simulink library "HY_General_Library"  (R2018b)
settings: Solver=ode45  StartTime=0.0  StopTime=10.0  RelTol=1e-3  EnableMultiTasking=on
undefined symbols (not defined in the file or in its folder): dT, Slope1, Slope2
libraries: simulink x63, $bdroot x4
(part 1 of 5)
settings Model: Creator=zhangzhi35  LastModifiedBy=xuhongjiang01
settings DataIOCC: LimitDataPoints=on  SaveFormat=Array
settings OptimizationCC: LifeSpan=inf
settings DebuggingCC: SolverPrmCheckMsg=warning  SFUnexpectedBacktrackingDiag=warning  SFNoUnconditionalDefaultTransitionDiag=warning  SFExecutionAtInitializationDiag=none
settings HardwareCC: ProdBitPerPointer=32  ProdBitPerSizeT=32  ProdBitPerPtrDiffT=32  ProdLargestAtomicFloat=None  ProdIntDivRoundTo=Undefined  ProdEndianess=Unspecified  ProdWordSize=32  ProdHWDeviceType=32-bit Generic
settings ModelReferenceCC: PropagateSignalLabelsOutOfModel=off
settings SFSimCC: SimUseLocalCustomCode=off
settings RTWCC: RTWUseLocalCustomCode=off
settings CodeAppCC: StateflowObjectComments=on
settings GRTTargetCC: TargetLangStandard=C89/C90 (ANSI)  GeneratePreprocessorConditionals=Disable all
settings ConfigComp: CovMetricSettings=dw  CovHtmlReporting=on  CovSaveCumulativeToWorkspaceVar=on  CovSaveSingleToWorkspaceVar=on  CovExternalEMLEnable=off  CovSFcnEnable=off

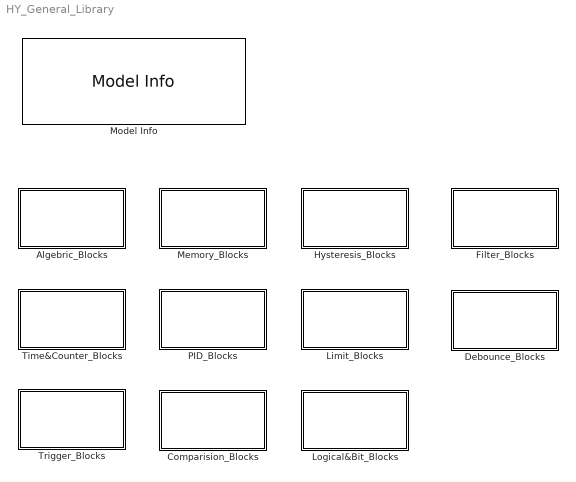
== system HY_General_Library ==
  Algebric_Blocks : Subsystem
      mask Display:
      | color('magenta')
      | fprintf('ALGEBRIC\nBLOCKS')
  Comparision_Blocks : Subsystem
      mask Display:
      | color('magenta')
      | fprintf('COMPARISION\nBLOCKS')
  Debounce_Blocks : Subsystem
      mask Display:
      | color('magenta')
      | fprintf('DEBOUNCE\nBLOCKS')
  Filter_Blocks : Subsystem
      mask Display:
      | color('magenta')
      | fprintf('FILTER\nBLOCKS')
  Hysteresis_Blocks : Subsystem
      mask Display:
      | color('magenta')
      | fprintf('HYSTERESIS\nBLOCKS')
  Limit_Blocks : Subsystem
      mask Display:
      | color('magenta')
      | fprintf('LIMIT\nBLOCKS')
  Logical&Bit_Blocks : Subsystem
      mask Display:
      | color('magenta')
      | fprintf('LOGIC&BIT\nBLOCKS')
  Memory_Blocks : Subsystem
      mask Display:
      | color('magenta')
      | fprintf('MEMORY\nBLOCKS')
  Model Info : simulink/Model-Wide Utilities/Model Info  Frame=on  DisplayStringWithTags=|  HorizontalTextAlignment=Left  LeftAlignmentValue=0.02
      | ModelName:     %<ModelName>                   
      |   Creator:             %<Creator>
      |   Created Date:   %<Created>
      |   ModelVersion:   %<ModelVersion>
      |   LastModifier:     %<LastModifiedBy>
      |   Modified Date:   %<LastModificationDate>
  PID_Blocks : Subsystem
      mask Display:
      | color('magenta')
      | fprintf('PID\nBLOCKS')
  Time&Counter_Blocks : Subsystem
      mask Display:
      | color('magenta')
      | fprintf('TIME&COUNTER\nBLOCKS')
  Trigger_Blocks : Subsystem
      mask Display:
      | color('magenta')
      | fprintf('TRIGGER\nBLOCKS')

== system HY_General_Library/Algebric_Blocks ==
  DIVIDE : Subsystem  mask(DIVIDE){MinRange=1e-5}
      mask prompts: MinRange "Smallest allowed value to divide by"
      mask help:
      | HY Library for Function Development
      |
      | Divides two inputs with divide by zero protection.
      |
      | The minimal value to divide by is set by the project lead and may not be changed.
      |
      | When abs(second input) is less than the specified MinRange,
      | then the second input is substituted by MinRange or -MinRange for negative values.
      mask init:
      | val=get_param(gcb,'MinRange');
      | if strcmp(val,'0')
      |     val = '1e-5';
      |     set_param(gcb,'MinRange',val);
      |     errordlg('Invalid setting in block DIVIDE_Protect');  
      | end
      mask Display:
      | port_label('input',1,'×');
      | port_label('input',2,'÷')
      | color('magenta');
      | text(1,0,'HY','horizontalAlignment','right','verticalAlignment','bottom');
  TrqPwr_Cnv : Subsystem  mask(TrqPwr_Cnv){CnvType=TrqSpd --> Pwr, Trq2Pwr=boolean(1)}
      mask prompts: CnvType "转换类型:"; Trq2Pwr "Mask Parameter 2:"
      mask help:
      | 皓耘功能开发库
      |
      | 扭矩功率转换器
      |
      | 可在参数设置界面选择转换类型
      | P=TN/9550
      |
      | 输入/输出：
      | Spd：转速信号，单位RPM
      | Trq：扭矩，单位Nm
      | Pwr：功率，单位kW
      mask Help:
      | 1、功率扭矩计算速度，使用公式 N = P * 9550 / T
      | 2、功率速度计算扭矩，使用公式 T = P * 9550 / N
      | 3、扭矩速度计算功率，使用公式 P = T * N / 9550
      | 
      | 1与2可使用同一类型计算
      mask TypeOptions CnvType: TrqSpd --> Pwr | PwrSpd --> Trq | PwrTrq --> Spd
      mask Callback CnvType:
      | switch get_param(gcb,'CnvType')
      |     case 'TrqSpd --> Pwr'
      |         Trq2Pwr = 1;
      |     case 'PwrSpd --> Trq'
      |         Trq2Pwr = 0;
      |     case 'PwrTrq --> Spd'
      |         Trq2Pwr = 0;
      | end
      | set_param(gcb,'Trq2Pwr',['boolean(' num2str(Trq2Pwr) ')']);
      mask Display:
      | port_label('input',1,CnvType(1:3));
      | port_label('input',2,CnvType(4:6));
      | port_label('output',1,CnvType(end-2:end));
      | color('blue')
      | disp(CnvType, 'texmode','on')
      | color('magenta');
      | text(1,0,'HY','horizontalAlignment','right','verticalAlignment','bottom');
  Unit_Cnv : Subsystem  RTWFcnName=Unit_Cnv  RTWFileName=SEN_MDL_LIB  mask(Unit conversions){CnvType=km/h --> m/s, g=single(0.27778)}
      mask prompts: CnvType "Conversion Type:"; g "Mask Parameter 2:"
      mask help:
      | 皓耘功能开发库
      |
      | Conversions of units.
      settings: RTWFcnNameOpts=User specified  RTWFileNameOpts=User specified
      mask TypeOptions CnvType: rad --> deg | deg --> rad | pascal --> bar | bar --> pascal | kilopascal --> bar | bar --> kilopascal | min --> sec | sec --> min | hour --> sec | sec --> hour | km --> mile | mile --> km | km/h --> m/s | m/s --> km/h | rad/s --> rpm | rpm --> rad/s | xx --> kiloxx | kiloxx --> xx
      mask Callback CnvType:
      | switch get_param(gcb,'CnvType')
      |     case 'rad --> deg'
      |         g = 57.2958;
      |     case 'deg --> rad'
      |         g = 0.017453;
      |     case 'bar --> pascal'
      |         g=1e5;
      |     case 'pascal --> bar'
      |         g=1e-5;
      |     case 'bar --> kilopascal'
      |         g=100;
      |     case 'kilopascal --> bar'
      |         g=0.01;
      |     case 'min --> sec'
      |         g=60;
      |     case 'sec --> min'
      |         g=1/60;
      |     case 'hour --> sec'
      |         g=3600;
      |     case 'sec --> hour'
      |         g=1/3600;
      |     case 'km --> mile'
      |         g=1/1.6093;
      |     case 'mile --> km'
      |         g=1.6093;
      |     case 'km/h --> m/s'
      |         g=1000/3600;
      |     case 'm/s --> km/h'
      |         g=3.6;
      |     case 'rad/s --> rpm'
      |         g=60/(2*pi);
      |     case 'rpm --> rad/s'
      |         g=2*pi/60;
      |     case 'xx --> kiloxx'
      |         g=0.001;
      |     case 'kiloxx --> xx'
      |         g=1000;
      | end
      | set_param(gcb,'g',['single(' num2str(g) ')']);
      mask Display:
      | color('blue')
      | disp(CnvType, 'texmode','on')
      | color('magenta');
      | text(0.93,0,'HY','horizontalAlignment','right','verticalAlignment','bottom');

== system HY_General_Library/Comparision_Blocks ==
  Open_Interval : Subsystem  RTWFcnName=Open_Interval  RTWFileName=SEN_MDL_LIB  mask(Open_Interval){CompareType=L<u<H, sIndex=uint8(0)}
      mask prompts: CompareType "Comparision Type:"; sIndex "Switch Parameter"
      mask help:
      | 皓耘功能开发库
      |
      | 区间模块
      |
      | 输入:
      | H：上限阀值
      | u：信号输入
      | L：下限阀值
      |
      | 输出：
      | y：输出信号（布尔型）
      settings: MinAlgLoopOccurrences=on  RTWFcnNameOpts=User specified  RTWFileNameOpts=User specified
      mask TypeOptions CompareType: L<u<H | L≤x<H | L<x≤H | L≤x≤H
      mask Callback CompareType:
      | switch get_param(gcb,'CompareType')
      |     case 'L<u<H'
      |         sIndex = 0;
      |     case 'L≤x<H'
      |         sIndex = 1;
      |     case 'L<x≤H'
      |         sIndex = 2;
      |     case 'L≤x≤H'
      |         sIndex = 3;
      | end
      | set_param(gcb,'sIndex',['uint8(' num2str(sIndex) ')']);
      mask Display:
      | color('blue');
      | disp(CompareType, 'texmode','on');
      | color('black');
      | port_label('input',1,'H');
      | port_label('input',2,'u');
      | port_label('input',3,'L');
      | color('orange');
      | port_label('output',1,'y');
      | color('magenta');
      | text(1,0,'HY','horizontalAlignment','right','verticalAlignment','bottom');

== system HY_General_Library/Debounce_Blocks ==
  DebounceB : Subsystem  RTWFcnName=Debounce  RTWFileName=SEN_MDL_LIB  mask(DebounceB){InitialValue=0}
      mask prompts: InitialValue "初始输出值"
      mask help:
      | 皓耘功能开发库
      |
      | 开关信号防抖模块
      |
      | 输入：
      | u：     开关信号输入（布尔型）
      | TAct：  Active确认时间（浮点类型）
      | TDeact：Deactive激活确认时间（浮点类型）
      | dT：    模块运行单步时间（浮点类型）
      |
      | 输出：
      | y：     防抖处理后输出信号（布尔型）
      mask init:
      | val = get_param(gcb,'InitialValue');
      | if strcmp(val,'0')==0 && strcmp(val,'1')==0
      |     val = '0';
      |     set_param(gcb,'InitialValue',val);
      |     errordlg('This parameter can only be set to 0 or 1');  
      | end
      settings: RTWFcnNameOpts=User specified  RTWFileNameOpts=User specified
      mask Display:
      | color('orange');
      | port_label('input',1,'u');
      | port_label('output',1,'y');
      | color('black');
      | port_label('input',2,'TAct');
      | port_label('input',3,'TDeact');
      | port_label('input',4,'dT');
      | 
      | color('red')
      | plot([0.10 0.20 0.20],[0.55 0.55 0.75])
      | plot([0.20 0.22 0.22],[0.75 0.75 0.55])
      | plot([0.22 0.24 0.24],[0.55 0.55 0.75])
      | plot([0.24 0.26 0.26],[0.75 0.75 0.55])
      | plot([0.26 0.28 0.28],[0.55 0.55 0.75])
      | plot([0.28 0.70 0.70],[0.75 0.75 0.55])
      | plot([0.70 0.72 0.72],[0.55 0.55 0.75])
      | plot([0.72 0.74 0.74],[0.75 0.75 0.55])
      | plot([0.74 0.76 0.76],[0.55 0.55 0.75])
      | plot([0.76 0.78 0.78 0.90],[0.75 0.75 0.55 0.55])
      | plot([0.10 0.28 0.28],[0.25 0.25 0.45])
      | plot([0.28 0.78 0.78 0.90],[0.45 0.45 0.25 0.25])
      | color('black')
      | plot([0.20 0.27],[0.55 0.75])
      | plot([0.20 0.27],[0.75 0.55])
      | plot([0.70 0.78],[0.55 0.75])
      | plot([0.70 0.78],[0.75 0.55])
      | color('blue')
      | text(0.35,0.1,sprintf('InitVal=%s', char(val)));
      | color('magenta')
      | text(1,0,'HY','horizontalAlignment','right','verticalAlignment','bottom')
  DebounceJump : Subsystem  mask(DebounceJump){}
      mask help:
      | 皓耘功能开发库
      |
      | 信号跳变处理模块
      |
      | 输入信号与上一时刻输出值相差超过设定幅值开始计时，否则计时清零
      | 计时超过最大检查时间，输出当前值，否则，输出上一时刻值
      |
      | 输入：
      | u：    需处理信号
      | Thd：  信号跳变幅值
      | ChkTi：最大检查时间（秒）
      | dT：   模块运行单步时间（秒）
      |
      | 输出：
      | y：    处理后的信号
      mask Display:
      | color('magenta');
      | text(1,0,'HY','horizontalAlignment','right','verticalAlignment','bottom');
  Debounce_Cnt : Subsystem  RTWFcnName=Debounce  RTWFileName=SEN_MDL_LIB  mask(Debounce_Cnt){InitialValue=0}
      mask prompts: InitialValue "初始输出值"
      mask help:
      | 皓耘功能开发库
      |
      | 基于运行次数的开关信号防抖模块
      |
      | 输入：
      | u：     开关信号输入（布尔型）
      | ONCnt： ON延时次数（无符号整型）
      | OFFCnt：ON延时次数（无符号整型）
      |
      | 输出：
      | y：     防抖处理后输出信号（布尔型）
      mask init:
      | val = get_param(gcb,'InitialValue');
      | if strcmp(val,'0')==0 && strcmp(val,'1')==0
      |     val = '0';
      |     set_param(gcb,'InitialValue',val);
      |     errordlg('This parameter can only be set to 0 or 1');  
      | end
      settings: RTWFcnNameOpts=User specified  RTWFileNameOpts=User specified
      mask Display:
      | color('orange');
      | port_label('input',1,'u');
      | port_label('output',1,'y');
      | color('black');
      | port_label('input',2,'ONCnt');
      | port_label('input',3,'OFFCnt');
      | 
      | color('red')
      | plot([0.10 0.20 0.20],[0.55 0.55 0.75])
      | plot([0.20 0.22 0.22],[0.75 0.75 0.55])
      | plot([0.22 0.24 0.24],[0.55 0.55 0.75])
      | plot([0.24 0.26 0.26],[0.75 0.75 0.55])
      | plot([0.26 0.28 0.28],[0.55 0.55 0.75])
      | plot([0.28 0.70 0.70],[0.75 0.75 0.55])
      | plot([0.70 0.72 0.72],[0.55 0.55 0.75])
      | plot([0.72 0.74 0.74],[0.75 0.75 0.55])
      | plot([0.74 0.76 0.76],[0.55 0.55 0.75])
      | plot([0.76 0.78 0.78 0.90],[0.75 0.75 0.55 0.55])
      | plot([0.10 0.28 0.28],[0.25 0.25 0.45])
      | plot([0.28 0.78 0.78 0.90],[0.45 0.45 0.25 0.25])
      | color('black')
      | plot([0.20 0.27],[0.55 0.75])
      | plot([0.20 0.27],[0.75 0.55])
      | plot([0.70 0.78],[0.55 0.75])
      | plot([0.70 0.78],[0.75 0.55])
      | color('blue')
      | text(0.35,0.1,sprintf('InitVal=%s', char(val)));
      | color('magenta')
      | text(1,0,'HY','horizontalAlignment','right','verticalAlignment','bottom')
  Debounce_OBD_FCN : Subsystem  TreatAsAtomicUnit=on  mask(Debounce_OBD_FCN){}
      mask help:
      | 皓耘功能开发库
      |
      | ISO 14229 D.5  DTC-FaultDetectionCounter operation definition
      | 输入：
      | bErr        Error signal(s)  (i.e. vector of continuous test runs)
      | bRst        Reset flag  (true/false)
      | bEna        Enable flag (true/false)
      | FailThd     counter a value between 0 and 32767  (for each bErr signal)
      | RecThd      counter a value between 0 and -32768 (for each bErr signal)
      | IncrFail    increment Fault counter (>0) max 255 in timer ticks for each signal
      | DecrRec     decrement Recovery counter (<0) min -128 in timer ticks for each
      |             signal
      |
      | So Counters are in numbers of timer ticks of tiTaskA(=0.01);
      | E.g. if Increment counter is 5 and decrement counter -3 then
      | maximum fail and recovery times are:
      | 32767*0.01/5 = 65.534 sec and -32768*0.01/3 = 109.2267 sec at most
      |
      | Outputs :
      | bFailed testFailed  (Bit 0)
      |
      | Notes:
      | * Outputs are held when input bEna is disabled
      | * Due to Int16 instead of Int8 and Incr/Decr 5/-3 by default the above
      | mentioned ISO standard is somewhat changed.
      mask Display:
      | color('black');
      | plot([0.2,0.2],[0.1,0.9]);
      | plot([0.205,0.205],[0.1,0.9]);
      | plot([0.2,0.8],[0.8,0.8]);
      | plot([0.2,0.8],[0.65,0.65]);
      | plot([0.2,0.8],[0.45,0.45]);
      | plot([0.2,0.8],[0.25,0.25]);
      | plot([0.2,0.8],[0.1,0.1]);
      | port_label('input',1,'bErr');
      | port_label('input',2,'bRst');
      | port_label('input',3,'bEna');
      | port_label('input',4,'FailThd');
      | port_label('input',5,'RecThd');
      | port_label('input',6,'IncrFail');
      | port_label('input',7,'DecrRec');
      | port_label('output',1,'bFailed');
      | color('cyan');
      | plot([0.3,0.3],[0.1,0.9]);
      | plot([0.4,0.4],[0.1,0.9]);
      | plot([0.5,0.5],[0.1,0.9]);
      | color('orange');
      | plot([0.2,0.3,0.3,0.6,0.6,0.8],[0.85,0.85,0.8,0.8,0.85,0.85]);
      | plot([0.2,0.5,0.5,0.6,0.6,0.8],[0.7,0.7,0.65,0.65,0.7,0.7]);
      | color('blue');
      | plot([0.2,0.3,0.4,0.5,0.5,0.6,0.7,0.8],[0.45,0.55,0.35,0.35,0.45,0.45,0.6,0.6]);
      | color('red');
      | plot([0.2,0.7,0.7,0.8],[0.25,0.25,0.3,0.3]);
      | color('green');
      | plot([0.2,0.4,0.4,0.5,0.5,0.8],[0.1,0.1,0.15,0.15,0.1,0.1]);
      | 
      | color('magenta')
      | text(1,0,'HY','horizontalAlignment','right','verticalAlignment','bottom')
  Debounce_OBD_FCN_St : Subsystem  TreatAsAtomicUnit=on  mask(Debounce_OBD_FCN_St){}
      mask help:
      | 皓耘功能开发库
      |
      | ISO 14229 D.5  DTC-FaultDetectionCounter operation definition
      | Inputs:
      | bErr        Error signal(s)  (i.e. vector of continuous test runs)
      | bRst        Reset flag  (true/false)
      | bEna        Enable flag (true/false)
      | FailThd     counter a value between 0 and 32767  (for each bErr signal)
      | RecThd      counter a value between 0 and -32768 (for each bErr signal)
      | IncrFail    increment Fault counter (>0) max 255 in timer ticks for each signal
      | DecrRec     decrement Recovery counter (<0) min -128 in timer ticks for each
      |             signal
      | bWIndAcv    Warm indictior active
      |
      | So Counters are in numbers of timer ticks of tiTaskA(=0.01);
      | E.g. if Increment counter is 5 and decrement counter -3 then
      | maximum fail and recovery times are:
      | 32767*0.01/5 = 65.534 sec and -32768*0.01/3 = 109.2267 sec at most
      |
      | Outputs :
      | bFailed     testFailed  (Bit 0)
      | bErrCfrm    confirmedDTC (Bit 3)
      | stDgo       (nach definition)
      | bNCompl     test not Completed (bit 6)
      |
      | Notes:
      | * Outputs are held when input bEna is disabled
      | * Due to Int16 instead of Int8 and Incr/Decr 5/-3 by default the above
      | mentioned ISO standard is somewhat changed.
      mask Display:
      | color('black');
      | plot([0.2,0.2],[0.1,0.9]);
      | plot([0.205,0.205],[0.1,0.9]);
      | plot([0.2,0.8],[0.8,0.8]);
      | plot([0.2,0.8],[0.65,0.65]);
      | plot([0.2,0.8],[0.45,0.45]);
      | plot([0.2,0.8],[0.25,0.25]);
      | plot([0.2,0.8],[0.1,0.1]);
      | port_label('input',1,'bErr');
      | port_label('input',2,'bRst');
      | port_label('input',3,'bEna');
      | port_label('input',4,'FailThd');
      | port_label('input',5,'RecThd');
      | port_label('input',6,'IncrFail');
      | port_label('input',7,'DecrRec');
      | port_label('input',8,'bWIndAcv');
      | port_label('output',1,'bFailed');
      | port_label('output',2,'bNCompl');
      | port_label('output',3,'bErrCfm');
      | port_label('output',4,'stDgo');
      | color('cyan');
      | plot([0.3,0.3],[0.1,0.9]);
      | plot([0.4,0.4],[0.1,0.9]);
      | plot([0.5,0.5],[0.1,0.9]);
      | color('orange');
      | plot([0.2,0.3,0.3,0.6,0.6,0.8],[0.85,0.85,0.8,0.8,0.85,0.85]);
      | plot([0.2,0.5,0.5,0.6,0.6,0.8],[0.7,0.7,0.65,0.65,0.7,0.7]);
      | color('blue');
      | plot([0.2,0.3,0.4,0.5,0.5,0.6,0.7,0.8],[0.45,0.55,0.35,0.35,0.45,0.45,0.6,0.6]);
      | color('red');
      | plot([0.2,0.7,0.7,0.8],[0.25,0.25,0.3,0.3]);
      | color('green');
      | plot([0.2,0.4,0.4,0.5,0.5,0.8],[0.1,0.1,0.15,0.15,0.1,0.1]);
      | 
      | color('magenta')
      | text(1,0,'HY','horizontalAlignment','right','verticalAlignment','bottom')
  FaultDebounce : Subsystem  TreatAsAtomicUnit=on  mask(FaultDebounce){}
      mask help:
      | 皓耘功能开发库
      |
      | 故障诊断确认模块
      |
      | 此模块为连续诊断模块，bErr上升沿或下降沿触发时，直接清零计数
      | 某状态计数值在模块每次运行时加1，到达阀值后输出诊断结果，清零计数
      | 任一状态诊断过程中，另一状态的诊断计数保持清零
      | 诊断确认使能标志为False时，直接输出bErr状态
      |
      | 输入：
      | bErr：      故障标志（布尔型）
      | FailCntThd：故障确认计数阀值 （无符号整型）
      | RecCntThd： 故障恢复计数阀值 （无符号整型）
      | bEna：      诊断确认使能标志 （布尔型）
      | bRst：      计数清零使能标志（布尔型）
      |
      | 输出：
      | bFailed：   诊断后故障标志（布尔型）
      mask Help: 此模块为连续诊断模块，bErr上升沿或下降沿触发时，直接清零计数
      mask Display:
      | color('magenta')
      | text(1,0,'HY','horizontalAlignment','right','verticalAlignment','bottom')

== system HY_General_Library/Filter_Blocks ==
  Average_LPF : Subsystem  RTWFcnName=Average_LPF  RTWFileName=SEN_MDL_LIB  mask(Average_LPF){SampleTime=-1}
      mask prompts: SampleTime "Sample time"
      mask help:
      | 皓耘功能开发库
      |
      | 均值滤波器
      |
      | 输入：
      | u:  待滤波信号
      | Nr: 滤波个数（2<=Nr<=20）
      |
      | 输出：
      | y:    滤波信号输出
      | SigOK:滤波输出信号可靠标志
      |
      | 滤波信号未达到Nr个数时，SigOK为False
      mask init:
      | tps=0.2:0.016:1;
      | in=[0.7500 
      | 	0.7500
      | 	0.8086
      |     0.8539
      |     0.8216
      |     0.7714
      |     0.6922
      |     0.6177
      |     0.6664
      |     0.6533
      |     0.7042
      |     0.7827
      |     0.8477
      |     0.8433
      |     0.8707
      |     0.7885
      |     0.6930
      |     0.6254
      |     0.6328
      |     0.6438
      |     0.7447
      |     0.7976
      |     0.8579
      |     0.8897
      |     0.8418
      |     0.7622
      |     0.6449
      |     0.6590
      |     0.5935
      |     0.7118
      |     0.7719
      |     0.8605
      |     0.8268
      |     0.8103
      |     0.8166
      |     0.7517
      |     0.6413
      |     0.6451
      |     0.6931
      |     0.7093
      |     0.7207
      |     0.8986
      |     0.7884
      |     0.8173
      |     0.8879
      |     0.6447
      |     0.7140
      |     0.6152
      |     0.6063
      |     0.7549
      |     0.7665];
      | 
      | out=[    0.2500
      |     0.2500
      |     0.2793
      |     0.3042
      |     0.3085
      |     0.3011
      |     0.2829
      |     0.2593
      |     0.2477
      |     0.2372
      |     0.2339
      |     0.2384
      |     0.2475
      |     0.2549
      |     0.2631
      |     0.2648
      |     0.2603
      |     0.2524
      |     0.2457
      |     0.2404
      |     0.2406
      |     0.2433
      |     0.2485
      |     0.2547
      |     0.2583
      |     0.2584
      |     0.2541
      |     0.2506
      |     0.2449
      |     0.2438
      |     0.2447
      |     0.2485
      |     0.2509
      |     0.2527
      |     0.2546
      |     0.2545
      |     0.2514
      |     0.2485
      |     0.2470
      |     0.2461
      |     0.2454
      |     0.2492
      |     0.2501
      |     0.2517
      |     0.2548
      |     0.2523
      |     0.2515
      |     0.2486
      |     0.2456
      |     0.2458
      |     0.2462];
      settings: AttributesFormatString=Average_LPF  RTWFcnNameOpts=User specified  RTWFileNameOpts=User specified
      mask Display:
      | color('blue')
      | plot(tps(1:end-10),in(1:end-10));
      | plot(tps(1:end-10),out(1:end-10)+0.1);
      | text(0.5,0.95,'In');
      | text(0.35,0.45,'Average(In)');
      | color('magenta');
      | text(1,0,'HY','horizontalAlignment','right','verticalAlignment','bottom');
  DT1 : Subsystem  RTWFcnName=DT1  RTWFileName=SEN_MDL_LIB  mask(DT1){}
      mask help:
      | HY Library for Function Development
      |
      | Differential-Element with 1st order delay
      settings: AttributesFormatString=DT1  RTWFcnNameOpts=User specified  RTWFileNameOpts=User specified
      mask Display:
      | color('black');
      | plot(0,0,100,100,[78,80,78,80,20,20,22,20,19],[17,20,23,20,20,93,91,93,91],[82,16],[70,70]);
      | color('blue');
      | plot([78,67,58,50,43,37,31,26,23,21,20],[20,21,22,25,30,36,45,55,60,65,67]);
      | plot([10,13,13,16,16,18],[4,4,15,15,4,4]);
      | disp('DT1');
      | color('orange');
      | port_label('input',3,'R','texmode','on');
      | color('black');
      | port_label('input',1,'u','texmode','on');
      | port_label('input',2,'RV','texmode','on');
      | port_label('input',4,'T','texmode','on');
      | port_label('input',5,'dT','texmode','on');
      | port_label('output',1,'y');
      | 
      | color('magenta');
      | text(100,0,'HY','horizontalAlignment','right','verticalAlignment','bottom');
  LPF1_K : Subsystem  mask(LPF1_K){}
      mask help:
      | 皓耘功能开发库
      |
      | 一阶低通滤波器（基于系数）
      |
      | 输入
      | u: 待滤波信号
      | R: 滤波器复位标志
      | RV:滤波器复位输出值
      | K: 滤波系数 (0 <= K <=1 )
      |
      | 输出
      | y: 滤波信号输出
      |
      |    y(n) = K*u(n) + (1-K)*y(n-1) (0<=k<=1)
      settings: AttributesFormatString=LPF1_K
      mask Display:
      | color('black');
      | port_label('input',1,'u');
      | port_label('input',2,'K');
      | port_label('output',1,'y');
      | plot([0.2,0.8],[0.2,0.2]);
      | plot([0.2,0.2],[0.2,0.8]);
      | plot([0.2,0.3],[0.65,0.65]);
      | plot([0.35,0.45],[0.65,0.65]);
      | plot([0.5,0.6],[0.65,0.65]);
      | plot([0.65,0.75],[0.65,0.65]);
      | plot([0.75,0.8,0.75],[0.22,0.2,0.18]);
      | plot([0.18,0.2,0.22],[0.75,0.8,0.75])
      | color('blue');
      | plot([0:0.01:1]*0.55+0.20,(1-exp(-8*[0:0.01:1]))*0.45+0.20);
      | text(0.5,0.45,'K');
      | color('magenta');
      | text(1,0,'HY','horizontalAlignment','right','verticalAlignment','bottom');
  LPF1_K_R : Subsystem  mask(LPF1_K_R){}
      mask help:
      | 皓耘功能开发库
      |
      | 一阶低通滤波器带复位（基于系数）
      |
      | 输入：
      | u: 待滤波信号
      | R: 复位使能
      | RV:复位值
      | K:滤波系数 (0 <= K <=1 )
      |
      | 输出：
      | y: 滤波信号输出
      |
      |
      | if R=1
      |    y=RV
      | else
      |    y(n) = K*u(n) + (1-K)*y(n-1) (0<=k<=1)
      settings: AttributesFormatString=LPF1_K_R
      mask Help:
      | if R=1
      |    y=RV
      | else
      |    y(n) = K*u(n) + (1-K)*y(n-1) (0<=k<=1)
      mask Display:
      | color('orange');
      | port_label('input',3,'R');
      | color('black');
      | port_label('input',1,'u');
      | port_label('input',2,'RV');
      | port_label('input',4,'K');
      | port_label('output',1,'y');
      | plot([0.2,0.8],[0.2,0.2]);
      | plot([0.2,0.2],[0.2,0.8]);
      | plot([0.2,0.3],[0.65,0.65]);
      | plot([0.35,0.45],[0.65,0.65]);
      | plot([0.5,0.6],[0.65,0.65]);
      | plot([0.65,0.75],[0.65,0.65]);
      | plot([0.75,0.8,0.75],[0.22,0.2,0.18]);
      | plot([0.18,0.2,0.22],[0.75,0.8,0.75])
      | color('blue');
      | plot([0:0.01:1]*0.55+0.20,(1-exp(-8*[0:0.01:1]))*0.45+0.20);
      | text(0.5,0.45,'K');
      | color('magenta');
      | text(1,0,'HY','horizontalAlignment','right','verticalAlignment','bottom');
  LPF1_T : Subsystem  mask(LPF1_T){}
      mask help:
      | 皓耘功能开发库
      |
      | 一阶低通滤波器（基于时间）
      |
      | 输入：
      | u: 待滤波信号
      | T: 滤波时间
      | dT:采样周期 (dT > 0)
      |
      | 输出：
      | y: 滤波信号输出
      |
      | y(n) = K*u(n) + (1-K)*y(n-1)
      | K = dT/T  (0<k<=1)
      settings: AttributesFormatString=LPF1_T
      mask Display:
      | color('black');
      | port_label('output',1,'y');
      | port_label('input',1,'u');
      | port_label('input',2,'T');
      | port_label('input',3,'dT');
      | plot([0.2,0.8],[0.2,0.2]);
      | plot([0.2,0.2],[0.2,0.8]);
      | plot([0.2,0.3],[0.65,0.65]);
      | plot([0.35,0.45],[0.65,0.65]);
      | plot([0.5,0.6],[0.65,0.65]);
      | plot([0.65,0.75],[0.65,0.65]);
      | plot([0.75,0.8,0.75],[0.22,0.2,0.18]);
      | plot([0.18,0.2,0.22],[0.75,0.8,0.75])
      | color('blue');
      | plot([0:0.01:1]*0.55+0.20,(1-exp(-8*[0:0.01:1]))*0.45+0.20);
      | text(0.5,0.45,'T');
      | color('magenta');
      | text(1,0,'HY','horizontalAlignment','right','verticalAlignment','bottom');
  LPF1_T_R : Subsystem  mask(LPF1_T_R){}
      mask help:
      | 皓耘功能开发库
      |
      | 一阶低通滤波器带复位（基于时间）
      |
      | 输入：
      | u: 待滤波信号
      | R: 复位使能
      | RV:复位值
      | T: 滤波时间
      | dT:采样周期 (dT > 0)
      |
      | 输出：
      | y: 滤波信号输出
      |
      | if R=1
      |    y=RV
      | else
      |    y(n) = K*u(n) + (1-K)*y(n-1)
      |    K = dT/T  (0<k<=1)
      settings: AttributesFormatString=LPF1_T_R
      mask Help:
      | if R=1
      |    y=RV
      | else
      |    y(n) = K*u(n) + (1-K)*y(n-1)
      |    K = dT/T  (0<k<=1)
      mask Display:
      | color('orange');
      | port_label('input',3,'R');
      | color('black');
      | port_label('input',1,'u');
      | port_label('input',2,'RV');
      | port_label('input',4,'T');
      | port_label('input',5,'dT');
      | port_label('output',1,'y');
      | plot([0.2,0.8],[0.2,0.2]);
      | plot([0.2,0.2],[0.2,0.8]);
      | plot([0.2,0.3],[0.65,0.65]);
      | plot([0.35,0.45],[0.65,0.65]);
      | plot([0.5,0.6],[0.65,0.65]);
      | plot([0.65,0.75],[0.65,0.65]);
      | plot([0.75,0.8,0.75],[0.22,0.2,0.18]);
      | plot([0.18,0.2,0.22],[0.75,0.8,0.75])
      | color('blue');
      | plot([0:0.01:1]*0.55+0.20,(1-exp(-8*[0:0.01:1]))*0.45+0.20);
      | text(0.5,0.45,'T');
      | 
      | color('magenta');
      | text(1,0,'HY','horizontalAlignment','right','verticalAlignment','bottom');
  LPF2_T_d_R : Subsystem  RTWFcnName=LPF2_T_d_ExtIni  RTWFileName=SEN_MDL_LIB  mask(LPF2_T_d_R){DataType=Inherit: Inherit via back propagation}
      mask prompts: DataType "Signal data type"
      mask help:
      | HY Library for Function Development
      |
      | Low pass filter, 2nd order implementation.
      |
      | Input signal is passed from port 'In'.
      | Time constant is passed from port 'T', unit is 'second'.
      | Damping factor is passed from port 'd'.
      | Sample time is passed from port 'dT', unit is 'second'. Sample time must not be 0.
      |
      | Simulink Standard Model Library.
      settings: AttributesFormatString=LPF2_T_d_R  RTWFcnNameOpts=User specified  RTWFileNameOpts=User specified
      mask Help:
      | Low pass filter, 2nd order implementation.
      | Input signal is passed from port 'In'.
      | Time constant is passed from port 'T'.
      | Damping factor is passed from port 'd'.
      | Sample time is passed from port 'dT'. Sample time must not be 0.
      mask Display:
      | color('black');
      | plot([0.15,0.85],[0.15 0.15]);
      | plot([0.15 0.15000001],[0.15 0.85]);
      | color('blue');
      | plot([0:0.01:1]*.68+.15,(1-exp(-15*0.5*[0:0.01:1]).*sin(sqrt(1-0.5^2)*15*[0:0.01:1]+atan(sqrt(1-0.5^2)/0.5))/sqrt(1-0.5^2))*.55+.15);
      | disp('LPF2');
      | plot([0.1,0.15,0.15,0.2,0.2,0.25],[0.05,0.05,0.12,0.12,0.05,0.05]);
      | color('black');
      | plot([0.16 0.19],[.7 .7],[0.23 0.26],[.7 .7],[0.30 0.33],[.7 .7],[0.37 0.40],[.7 .7],[0.44 0.47],[.7 .7],[0.51 0.54],[.7 .7],[0.58 0.61],[.7 .7]);
      | color('orange');
      | port_label('input',3,'R','texmode','on');
      | color('black');
      | port_label('input',1,'u','texmode','on');
      | port_label('input',2,'RV','texmode','on');
      | port_label('input',4,'d','texmode','on');
      | port_label('input',5,'T','texmode','on');
      | port_label('input',6,'dT','texmode','on');
      | port_label('output',1,'y','texmode','on');
      | 
      | color('magenta');
      | text(1,0,'HY','horizontalAlignment','right','verticalAlignment','bottom');

== system HY_General_Library/Hysteresis_Blocks ==
  HysteresisA : Subsystem  mask(HysteresisA){InitialValue=0}
      mask prompts: InitialValue "初始输出值"
      mask help:
      | 皓耘功能开发库
      | 正打开回滞器
      |
      | 输入：
      | u:    输入信号
      | ON:   ON阈值
      | OFF:  OFF阈值
      | IV：初始输出状态
      |
      | 输出：
      | y:    开关输出
      |
      | 当 u ≥ ON, 输出TRUE
      | If当u < OFF, 输出FALSE
      | 否则保持前一时刻状态
      |
      | 注意：
      | InitVal在参数界面设置
      | ON阈值需要大于OFF阈值
      mask init:
      | val=get_param(gcb,'InitialValue');
      | if strcmp(val,'0')==0 && strcmp(val,'1')==0
      |     val = '0';
      |     set_param(gcb,'InitialValue',val);
      |     errordlg('This parameter can only be set to 0 or 1');  
      | end
      settings: AttributesFormatString=Hysteresis
      mask Help:
      | 当 u ≥ ON, 输出TRUE
      | If当u < OFF, 输出FALSE
      | 否则保持前一时刻状态
      | 
      | 注意：
      | InitVal在参数界面设置
      | ON阈值需要大于OFF阈值
      mask Display:
      | color('orange');
      | port_label('output',1,'y');
      | color('black');
      | port_label('input',1,'ON');
      | port_label('input',2,'u');
      | port_label('input',3,'OFF');
      | color('blue');
      | plot([0.25 0.65 0.65],[0.2 0.2 0.8], ...
      |      [0.35 0.35 0.75],[0.2 0.8 0.8],...
      |      [0.32 0.35 0.38],[0.50 0.45 0.50],...
      |      [0.62 0.65 0.68],[0.45 0.5 0.45]);
      | text(0.67,0.6,'ON');
      | text(0.14,0.6,'OFF');
      | text(0.30,0.1,sprintf('InitVal = %s', char(val)));
      | color('magenta');
      | text(1,0,'HY','horizontalAlignment','right','verticalAlignment','bottom');
  HysteresisB : Subsystem  mask(HysteresisB){InitialValue=0}
      mask prompts: InitialValue "初始输出值"
      mask help:
      | 皓耘功能开发库
      |
      | 正关闭回滞器
      |
      | 当 u ≥ OFF, 输出False
      | 当u < ON, 输出True
      | 否则保持前一时刻状态
      |
      | 输入：
      | u:    输入信号
      | ON:   ON阈值
      | OFF:  OFF阈值
      |
      | 输出：
      | y:    开关输出
      mask init:
      | val=get_param(gcb,'InitialValue');
      | if strcmp(val,'0')==0 && strcmp(val,'1')==0
      |     val = '0';
      |     set_param(gcb,'InitialValue',val);
      |     errordlg('This parameter can only be set to 0 or 1');  
      | end
      settings: AttributesFormatString=Hysteresis
      mask Help:
      | 当 u ≥ OFF, 输出False
      | 当u < ON, 输出True
      | 否则保持前一时刻状态
      | 
      | 注意：
      | InitVal在参数界面设置
      | OFF阈值需要大于ON阈值
      mask Display:
      | color('orange');
      | port_label('output',1,'y');
      | color('black');
      | port_label('input',1,'OFF');
      | port_label('input',2,'u');
      | port_label('input',3,'ON');
      | color('blue');
      | plot([0.25 0.65 0.65],[0.8 0.8 0.2], ...
      |      [0.35 0.35 0.75],[0.8 0.2 0.2],...
      |      [0.32 0.35 0.38],[0.45 0.5 0.45],...
      |      [0.62 0.65 0.68],[0.50 0.45 0.5]);
      | text(0.68,0.6,'OFF');
      | text(0.16,0.6,'ON');
      | text(0.30,0.1,sprintf('InitVal = %s', char(val)));
      | color('magenta');
      | text(1,0,'HY','horizontalAlignment','right','verticalAlignment','bottom');

== system HY_General_Library/Limit_Blocks ==
  GrandientLimiter : Subsystem  mask(GrandientLimiter){}
      mask help:
      | HY Library for Function Development
      |
      | GrandientLimiter with reset.
      |
      | The output value is limited in its gradient to the last input value. The maximum valid difference is LU, the minimum valid difference is LD.
      | LD and LL have to be given with respect to sample time dT.
      |
      | inputs:
      | TV  - target value
      | BV  - base value
      | R   - reset block and forward RV to output signal
      | RV  - reset value
      | LU  - upper limit for gradient
      | LL  - lower limit for gradient
      | dT  - sample time for gradient calculation
      |
      | output:
      | y   - limited gradient
      mask Display:
      | plot([0.3,0.6],[0.5,0.5]);
      | plot([0.45,0.45],[0.2,0.8]);
      | plot([0.55,0.6,0.55],[0.53,0.5,0.47]);
      | plot([0.48,0.45,0.42],[0.75,0.8,0.75]);
      | color('blue');
      | plot([0.3,0.35,0.55,0.6],[0.3,0.3,0.7,0.7]);
      | 
      | color('magenta');
      | text(1,0,'HY','horizontalAlignment','right','verticalAlignment','bottom');
  LIMIT : Subsystem  Description=""  mask(LIMIT){}
      mask help:
      | 皓耘功能开发库
      |
      | 数值限制器
      |
      | 输入信号将被限制在最大最小允许范围之间
      |
      | 输入：
      | Max：最大允许值
      | Min：最小允许值
      | u：待处理信号
      |
      | 输出：
      | y：处理后输出值
      mask Display:
      | color('black');
      | plot([0.22,0.8],[0.5,0.5]);
      | plot([0.5,0.5],[0.2,0.8]);
      | plot([0.75,0.8,0.75],[0.53,0.5,0.46]);
      | plot([0.54,0.5,0.47],[0.76,0.8,0.76]);
      | color('blue');
      | plot([0.23,0.32,0.71,0.78],[0.3,0.3,0.7,0.7]);
      | 
      | color('magenta');
      | text(1,0,'HY','horizontalAlignment','right','verticalAlignment','bottom');
  Limit_Flag : Subsystem  Description=""  mask(Limit_Flag){}
      mask help:
      | 皓耘功能开发库
      |
      | 数值限制器（带标志）
      |
      | 输入信号将被限制在最大最小允许范围之间
      |
      | 输入：
      | Max：最大允许值
      | Min：最小允许值
      | u：待处理信号
      |
      | 输出：
      | y：处理后输出值
      | bMax：输入信号超上限标志
      | bMin：输入信号超下限标志
      mask Display:
      | color('black');
      | plot([0.22,0.7],[0.5,0.5]);
      | plot([0.45,0.45],[0.2,0.8]);
      | plot([0.65,0.7,0.65],[0.53,0.5,0.46]);
      | plot([0.43,0.45,0.48],[0.76,0.8,0.76]);
      | color('blue');
      | plot([0.23,0.32,0.6,0.7],[0.3,0.3,0.7,0.7]);
      | 
      | color('magenta');
      | text(1,0,'HY','horizontalAlignment','right','verticalAlignment','bottom');
  RateLimit_R : Subsystem  mask(RaterLimit_R){}
      mask help:
      | HY Library for Function Development
      |
      | RateLimit with reset.
      |
      | inputs:
      | u  - target value
      | R   - reset flag
      | RV  - reset value
      | Inc  - increase rate
      | Dec  - decrease rate
      | dT  - sample time
      |
      | output:
      | y   - limited gradient
      |
      | Apply change rate limit to input u, so that y(n) will be limited within [y(n-1)+Inc*dT, y(n-1)+Dec*dT].
      | Output will be reset to inital value (inport RV) when reset given TRUE (inport R).
      |
      | Note:
      |     Inc shall be positive while Dec shall be negative.
      settings: AttributesFormatString=RateLimit_R
      mask Display:
      | color('orange');
      | port_label('input',4,'R');
      | color('black');
      | port_label('input',1,'u');
      | port_label('input',2,'Inc');
      | port_label('input',3,'Dec');
      | port_label('input',5,'RV');
      | port_label('input',6,'dT');
      | port_label('output',1,'y');
      | plot([0.2,0.8],[0.5,0.5]);
      | plot([0.5,0.5],[0.2,0.8]);
      | plot([0.75,0.8,0.75],[0.53,0.5,0.47]);
      | plot([0.53,0.5,0.47],[0.75,0.8,0.75]);
      | color('blue');
      | plot([0.2,0.3,0.7,0.8],[0.3,0.3,0.7,0.7]);
      | 
      | color('magenta');
      | text(1,0,'HY','horizontalAlignment','right','verticalAlignment','bottom');

== system HY_General_Library/Logical&Bit_Blocks ==
  Extract_16bit : Subsystem  RTWFcnName=Extract_16bit  RTWFileName=SEN_MDL_LIB  mask(Extract_16bit){}
      mask help:
      | 皓耘功能开发库
      |
      | 16位提取器
      |
      | 输入：
      | U16In：16位无符号输入值
      |
      | 输出：
      | bitx：各位输出（布尔型）
      settings: AttributesFormatString=Extract_16bit  RTWFcnNameOpts=User specified  RTWFileNameOpts=User specified
      mask Display:
      | color('magenta');
      | text(1,0,'HY','horizontalAlignment','right','verticalAlignment','bottom');
  Extract_32bit : Subsystem  RTWFcnName=Extract_32bit  RTWFileName=SEN_MDL_LIB  mask(Extract_32bit){}
      mask help:
      | 皓耘功能开发库
      |
      | 32位提取器
      |
      | 输入：
      | U32In：32位无符号输入值
      |
      | 输出：
      | bitx：各位输出（布尔型）
      settings: AttributesFormatString=Extract_32bit  RTWFcnNameOpts=User specified  RTWFileNameOpts=User specified
      mask Display:
      | color('magenta');
      | text(1,0,'HY','horizontalAlignment','right','verticalAlignment','bottom');
  Extract_8bit : Subsystem  RTWFcnName=Extract_8bit  RTWFileName=SEN_MDL_LIB  mask(Extract_8bit){}
      mask help:
      | 皓耘功能开发库
      |
      | 8位提取器
      |
      | 输入：
      | U8In：8位无符号输入值
      |
      | 输出：
      | bitx：各位输出（布尔型）
      settings: AttributesFormatString=Extract_8bit  RTWFcnNameOpts=User specified  RTWFileNameOpts=User specified
      mask Display:
      | color('magenta');
      | text(1,0,'HY','horizontalAlignment','right','verticalAlignment','bottom');
  Integrate_16bit : Subsystem  RTWFcnName=Encoder_16bit_2_out  RTWFileName=SEN_MDL_LIB  mask(Integrate_16bit){}
      mask help:
      | 皓耘功能开发库
      |
      | 16位集成器
      |
      | 输入：
      | bitx：各位输入（布尔型）
      |
      | 输出：
      | U16Out：16位无符号输出值
      settings: AttributesFormatString=Integrate_16bit  RTWFcnNameOpts=User specified  RTWFileNameOpts=User specified
      mask Display:
      | color('magenta');
      | text(1,0,'HY','horizontalAlignment','right','verticalAlignment','bottom');
  Integrate_32bit : Subsystem  RTWFcnName=Encoder_32bit_2_out  RTWFileName=SEN_MDL_LIB  mask(Integrate_32bit){}
      mask help:
      | 皓耘功能开发库
      |
      | 32位集成器
      |
      | 输入：
      | bitx：各位输入（布尔型）
      |
      | 输出：
      | U32Out：32位无符号输出值
      settings: AttributesFormatString=Integrate_32bit  RTWFcnNameOpts=User specified  RTWFileNameOpts=User specified
      mask Display:
      | color('magenta');
      | text(1,0,'HY','horizontalAlignment','right','verticalAlignment','bottom');
  Integrate_8bit : Subsystem  RTWFcnName=Encoder_8bit_2_out  RTWFileName=SEN_MDL_LIB  mask(Integrate_8Bit){}
      mask help:
      | 皓耘功能开发库
      |
      | 8位集成器
      |
      | 输入：
      | bitx：各位输入（布尔型）
      |
      | 输出：
      | U8Out：8位无符号输出值
      settings: AttributesFormatString=Integrate_8bit  RTWFcnNameOpts=User specified  RTWFileNameOpts=User specified
      mask Display:
      | color('magenta');
      | text(1,0,'HY','horizontalAlignment','right','verticalAlignment','bottom');

== system HY_General_Library/Memory_Blocks ==
  EdgeBi : Subsystem  Tag=initial value = 0  mask(EdgeBi){}
      mask help:
      | 皓耘功能开发库
      |
      | 上升下降沿触发器
      |
      | 输入:
      | u - 逻辑输入信号 （True/False）
      |
      | 输出:
      | y - 输出信号 （True/False）
      |
      | 当输入由True变为False或由False变为Ture时，输出True，否则输出False
      mask init:
      | pos = get_param(gcb, 'Position');
      | x_c = (pos(3) - pos(1))/2;
      | y_c = (pos(4) - pos(2))/2;
      | y_c1 = y_c+5;
      | y_c2 = y_c-5;
      | sc1 = 10;
      | sc2 = 12;
      | sc3 = 4;
      | sc4 = 3;
      | sc5 = 3;
      mask Help: 当输入由True变为False或由False变为Ture时，输出True，否则输出False
      mask Display:
      | color('blue');
      | plot([0.15,0.5,0.5,0.85],[0.1,0.1,0.85,0.85]);
      | plot([0.35,0.5,0.65],[0.3,0.45,0.3]);
      | plot([0.35,0.5,0.65],[0.7,0.55,0.7]);
      | color('magenta');
      | text(1,0,'HY','horizontalAlignment','right','verticalAlignment','bottom');
  EdgeFalling : Subsystem  Tag=initial value = 0  mask(EdgeFalling){}
      mask help:
      | 皓耘功能开发库
      |
      | 下降沿触发器
      |
      | 输入:
      | u - 逻辑输入信号 （True/False）
      |
      | 输出:
      | y - 输出信号 （True/False）
      |
      | 当输入由True变为False时，输出True，否则输出False
      mask init:
      | pos = get_param(gcb, 'Position');
      | x_c = (pos(3) - pos(1))/2;
      | y_c = (pos(4) - pos(2))/2;
      | sc1 = 8;
      | sc2 = 8;
      | sc3 = 4;
      | sc4 = 3;
      | sc5 = 3;
      mask Help: 当输入由True变为False时，输出True，否则输出False
      mask Display:
      | color('blue');
      | plot([0.15,0.5,0.5,0.85],[0.85,0.85,0.1,0.1]);
      | plot([0.35,0.5,0.65],[0.6,0.45,0.6]);
      | color('magenta');
      | text(1,0,'HY','horizontalAlignment','right','verticalAlignment','bottom');
  EdgeRising : Subsystem  Tag=initial value = 0  mask(EdgeRising){}
      mask help:
      | 皓耘功能开发库
      |
      | 上升沿触发器
      |
      | 输入:
      | u - 逻辑输入信号 （True/False）
      |
      | 输出:
      | y - 输出信号 （True/False）
      |
      | 当输入由False变为True时，输出True，否则输出False
      mask init:
      | pos = get_param(gcb, 'Position');
      | x_c = (pos(3) - pos(1))/2;
      | y_c = (pos(4) - pos(2))/2;
      | sc1 = 8;
      | sc2 = 8;
      | sc3 = 4;
      | sc4 = 3;
      | sc5 = 3;
      mask Help: 当输入由False变为True时，输出True，否则输出False
      mask Display:
      | color('blue');
      | plot([0.15,0.5,0.5,0.85],[0.1,0.1,0.85,0.85]);
      | plot([0.35,0.5,0.65],[0.45,0.6,0.45]);
      | color('magenta');
      | text(1,0,'HY','horizontalAlignment','right','verticalAlignment','bottom');
  Mem : Subsystem  RTWFcnName=Mem  RTWFileName=SEN_MDL_LIB  mask(Mem){}
      mask help:
      | 皓耘功能开发库
      |
      | 信号保持器
      |
      | 输入：
      | u:待处理信号
      | Hld:保持使能
      |
      | 输出：
      | y:信号输出
      |
      |
      | 当Hld等于False时，信号输出等于实时信号
      | 当Hld等于True时，信号输出等于前一时刻信号输入
      settings: RTWFcnNameOpts=User specified  RTWFileNameOpts=User specified
      mask Help:
      | 当Hld等于False时，信号输出等于实时信号
      | 当Hld等于True时，信号输出等于前一时刻信号输入
      mask Display:
      | color('black')
      | port_label('input',1,'u');
      | port_label('output',1,'y');
      | color('orange')
      | port_label('input',2,'Hld');
      | 
      | color('blue')
      | plot([0.3 0.8 0.8 0.3 0.3],[0.2 0.2 0.8 0.8 0.6])
      | plot([0.2 0.3 0.4],[0.7 0.6 0.7])
      | plot([0.2 0.25 0.25 0.35 0.35 0.4],[0.3 0.3 0.5 0.5 0.3 0.3])
      | color('magenta');
      | text(1,0,'HY','horizontalAlignment','right','verticalAlignment','bottom');
  RS_FF : Subsystem  mask(RS_FF){InitialValue=0}
      mask prompts: InitialValue "Initial Value:"
      mask help:
      | 皓耘功能开发库
      |
      | 锁存器（正反输出）
      |
      | 输入：
      | S:锁存使能
      | R:复位使能
      | IV:初始化输出
      |
      | 输出：
      | Q:锁存器正输出
      | ~Q:锁存器反输出
      |
      | 初始化值在参数窗口设置
      | 复位使能优先级高于设置使能
      mask init:
      | val=get_param(gcb,'InitialValue');
      | if strcmp(val,'0')==0 && strcmp(val,'1')==0
      |     val = '0';
      |     set_param(gcb,'InitialValue',val);
      |     errordlg('This parameter can only be set to 0 or 1');  
      | end
      mask Help:
      | 初始化值在参数窗口设置
      | 复位使能优先级高于设置使能
      mask Display:
      | color('orange');
      | port_label('input',1,'S');
      | port_label('input',2,'R');
      | port_label('output',1,'Q');
      | port_label('output',2,'~Q');
      | 
      | color('blue');
      | disp('\fontsize{12}RS FF','texmode','on');
      | text(0.3,0.15,sprintf('InitVal=%s', char(val)));
      | 
      | color('magenta');
      | text(1,0,'HY','horizontalAlignment','right','verticalAlignment','bottom');
  RS_FF_IV : Subsystem  mask(RS_FF_IV){}
      mask help:
      | 皓耘功能开发库
      |
      | 锁存器初始值可调（反输出）
      |
      | 输入：
      | S:锁存使能
      | R:复位使能
      | IV:初始化输出
      |
      | 输出：
      | Q:锁存器正输出
      | ~Q:锁存器反输出
      |
      | 初始化值在端口输入设置
      | 复位使能优先级高于设置使能
      mask Help:
      | 初始化值在端口输入设置
      | 复位使能优先级高于设置使能
      mask Display:
      | color('orange');
      | port_label('input',1,'S');
      | port_label('input',2,'R');
      | port_label('input',3,'IV');
      | port_label('output',1,'Q');
      | port_label('output',2,'~Q');
      | 
      | color('blue');
      | disp('\fontsize{12}RS FF','texmode','on')
      | 
      | color('magenta');
      | text(1,0,'HY','horizontalAlignment','right','verticalAlignment','bottom');
  RS_FF_IV_Neg : Subsystem  mask(RS_FF_IV){}
      mask help:
      | 皓耘功能开发库
      |
      | 锁存器初始值可调（反输出）
      |
      | 输入：
      | S:锁存使能
      | R:复位使能
      | IV:初始化输出
      |
      | 输出：
      | ~Q:锁存器输出
      |
      | 初始化值在端口输入设置
      | 复位使能优先级高于设置使能
      mask Help:
      | 初始化值在端口输入设置
      | 复位使能优先级高于设置使能
      mask Display:
      | color('orange');
      | port_label('input',1,'S');
      | port_label('input',2,'R');
      | port_label('input',3,'IV');
      | port_label('output',1,'~Q');
      | 
      | color('blue');
      | disp('\fontsize{12}RS FF','texmode','on')
      | 
      | color('magenta');
      | text(1,0,'HY','horizontalAlignment','right','verticalAlignment','bottom');
  RS_FF_IV_Pos : Subsystem  mask(RS_FF_IV){}
      mask help:
      | 皓耘功能开发库
      |
      | 锁存器初始值可调（正输出）
      |
      | 输入：
      | S:锁存使能
      | R:复位使能
      | IV:初始化输出
      |
      | 输出：
      | Q:锁存器输出
      |
      | 初始化值在端口输入设置
      | 复位使能优先级高于设置使能
      mask Help:
      | 初始化值在端口输入设置
      | 复位使能优先级高于设置使能
      mask Display:
      | color('orange');
      | port_label('input',1,'S');
      | port_label('input',2,'R');
      | port_label('input',3,'IV');
      | port_label('output',1,'Q');
      | 
      | color('blue');
      | disp('\fontsize{12}RS FF','texmode','on');
      | 
      | color('magenta');
      | text(1,0,'HY','horizontalAlignment','right','verticalAlignment','bottom');
  RS_FF_Neg : Subsystem  mask(RS_FF){InitialValue=0}
      mask prompts: InitialValue "Initial Value:"
      mask help:
      | 皓耘功能开发库
      |
      | 锁存器（反输出）
      |
      | 输入：
      | S:锁存使能
      | R:复位使能
      | IV:初始化输出
      |
      | 输出：
      | ~Q:锁存器输出
      |
      | 初始化值在参数窗口设置
      | 复位使能优先级高于设置使能
      mask init:
      | val=get_param(gcb,'InitialValue');
      | if strcmp(val,'0')==0 && strcmp(val,'1')==0
      |     val = '0';
      |     set_param(gcb,'InitialValue',val);
      |     errordlg('This parameter can only be set to 0 or 1');  
      | end
      mask Help:
      | 初始化值在参数窗口设置
      | 复位使能优先级高于设置使能
      mask Display:
      | color('orange');
      | port_label('input',1,'S');
      | port_label('input',2,'R');
      | port_label('output',1,'~Q');
      | 
      | color('blue');
      | disp('\fontsize{12}RS FF','texmode','on');
      | text(0.30,0.15,sprintf('InitVal=%s', char(val)));
      | 
      | color('magenta');
      | text(1,0,'HY','horizontalAlignment','right','verticalAlignment','bottom');
  RS_FF_Pos : Subsystem  mask(RS_FF){InitialValue=0}
      mask prompts: InitialValue "Initial Value:"
      mask help:
      | 皓耘功能开发库
      |
      | 锁存器（正输出）
      |
      | 输入：
      | S:锁存使能
      | R:复位使能
      | IV:初始化输出
      |
      | 输出：
      | Q:锁存器输出
      |
      | 初始化值在参数窗口设置
      | 复位使能优先级高于设置使能
      mask init:
      | val=get_param(gcb,'InitialValue');
      | if strcmp(val,'0')==0 && strcmp(val,'1')==0
      |     val = '0';
      |     set_param(gcb,'InitialValue',val);
      |     errordlg('This parameter can only be set to 0 or 1');  
      | end
      mask Help:
      | 初始化值在参数窗口设置
      | 复位使能优先级高于设置使能
      mask Display:
      | color('orange');
      | port_label('input',1,'S');
      | port_label('input',2,'R');
      | port_label('output',1,'Q');
      | 
      | color('blue');
      | disp('\fontsize{12}RS FF','texmode','on');
      | text(0.30,0.15,sprintf('InitVal=%s', char(val)));
      | 
      | color('magenta');
      | text(1,0,'HY','horizontalAlignment','right','verticalAlignment','bottom');

== system HY_General_Library/PID_Blocks ==
  IncrementalPID : Subsystem  mask(INCPID){}
      mask help:
      | HY Library for Function Development
      | Incremental PID
      |
      | Inputs:
      | Err     ->Error
      | Kp      ->Propotion coefficient
      | Ki      ->Integral coefficient
      | Kd      ->Differential coefficient
      | ThdMax  ->Maximum output
      | ThdMin  ->Minimum output
      | R       ->Reset flag
      | RV      ->Reset value
      |
      | Output:
      | PIDOut     ->PIDOutput
      | POut       ->Proportion output
      | IOut       ->Integral output
      | DOut       ->Derivative output
      mask Display:
      | plot([0.35 0.8],[0.35 0.35]);
      | plot([0.35 0.35],[0.35 0.7]);
      | color('orange');
      | plot([0.35 0.73],[0.56 0.56]);
      | color('blue');
      | plot([0.4 0.44 0.45 0.46 0.48 0.52 0.56 0.60 0.65],[0.4 0.545 0.546 0.548 0.55 0.553 0.555 0.558 0.56]);
      | text(0.5,0.5,'Inc PID');
      | 
      | color('magenta');
      | text(1,0,'HY','horizontalAlignment','right','verticalAlignment','bottom');
  PositionPID : Subsystem  mask(POSPID){}
      mask help:
      | HY Library for Function Development
      | Position PID
      |
      | Inputs:
      | Err	 ->Error
      | CtrlPropVal  ->Propotion coefficient
      | CtrlIntgVal  ->Integral coefficient
      | CtrlDerivVal ->Differential coefficient
      | UpperSatLimd ->Upper Saturation Limit
      | FfEnaFlag    ->Feedforward Enable Flag
      | FfVal        ->Feedforward Value
      | ThdMax       ->Maximum output
      | ThdMin       ->Minimum output
      | Reset        ->Reset Integral Flag
      | ResetVal     ->Reset Integral Value
      | LowerSatLimd ->Lower Saturation Limit
      |
      | Output:
      | Output	 ->CtrlOutput
      mask Display:
      | plot([0.35 0.8],[0.35 0.35]);
      | plot([0.35 0.35],[0.35 0.7]);
      | color('orange');
      | plot([0.35 0.73],[0.56 0.56]);
      | color('blue');
      | plot([0.4 0.44 0.45 0.46 0.48 0.52 0.56 0.60 0.65],[0.4 0.545 0.546 0.548 0.55 0.553 0.555 0.558 0.56]);
      | text(0.5,0.5,'Pos PID');
      | 
      | color('magenta');
      | text(1,0,'HY','horizontalAlignment','right','verticalAlignment','bottom');
